simulink model "HD2_QArmTeleopClient"  (R2018a)
settings: Solver=ode1  StartTime=0.0  StopTime=inf  FixedStep=0.001  RelTol=1e-3  EnableMultiTasking=on
model workspace (MAT data in the model file):
  ErrTol = Simulink.Parameter
  ErrTol.Value = 0.0001
  ErrTol.DataType = 'auto'
  ErrTol.Dimensions = [1 1]
undefined symbols (not defined in the file): gcbh, Host, JPEG, video_display_show, Visualization
libraries: quarc_library x15, simulink x6, simulink_extras x3
settings Model: SimulationMode=external  ExtModeTrigDuration=10000  Creator=glai  LastModifiedBy=QuanserGraphics
settings SolverCC: PositivePriorityOrder=on
settings RTWCC: SystemTargetFile=quarc_win64.tlc  TemplateMakefile=quarc_default_tmf  Description=QUARC Win64 Target Using Toolchain  Toolchain=QUARC win64 | nmake (64-bit Windows)  BuildConfiguration=Faster Runs
settings CodeAppCC: StateflowObjectComments=on
settings STFCustomTargetCC: TargetLangStandard=C99 (ISO)  ConcurrentExecutionCompliant=on  UseToolchainInfoCompliant=on  SystemTargetFile=quarc_win64.tlc
settings GRTTargetCC: ParMdlRefBuildCompliant=off  CompOptLevelCompliant=off  CombineOutputUpdateFcns=off  MatFileLogging=off  CPPClassGenCompliant=off  GRTInterface=on  ExtMode=on  ExtModeMexFile=quarc_comm  ExtModeMexArgs='-w -d %d -uri %u -URI_SHMEM shmem://HD2_DRIVER_PY:0','tcpip://localhost:17005'
settings ConfigComp: CovMetricSettings=dswe

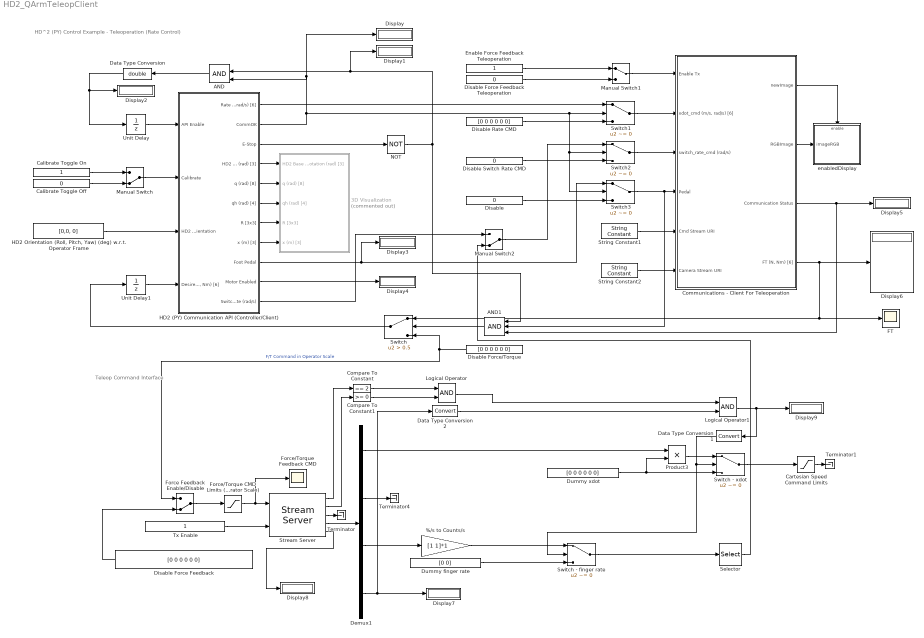
== system HD2_QArmTeleopClient ==
  note: HD^2 (PY) Control Example - Teleoperation (Rate Control)
  note: Teleop Command Interface
  %/s to Counts/s : Gain  Gain=[1 1]*1
  3D Visualization : Subsystem  Commented=on
  AND : Logic  IconShape=distinctive  AllPortsSameDT=off  OutDataTypeStr=boolean
  AND1 : Logic  Inputs=3  IconShape=distinctive  AllPortsSameDT=off  OutDataTypeStr=boolean
  Calibrate Toggle Off : Constant  Value=0
  Calibrate Toggle On : Constant
  Cartesian Speed Command Limits : Saturate  UpperLimit=[0.254 0.254 0.254 0.06 0.06 0.06]  LowerLimit=-1*[0.254 0.254 0.254 0.06 0.06 0.06]
  Communications - Client For Teleoperation : Subsystem
  Compare To Constant : simulink/Logic and Bit Operations/Compare To Constant  relop===  const=2  OutDataTypeStr=boolean
  Compare To Constant1 : simulink/Logic and Bit Operations/Compare To Constant  relop=>=  const=0  OutDataTypeStr=boolean
  Data Type Conversion : DataTypeConversion  OutDataTypeStr=double
  Data Type Conversion1 : DataTypeConversion
  Data Type Conversion2 : DataTypeConversion
  Demux1 : Demux  Outputs=[6 6 1 1]
  Disable : Constant  Value=0
  Disable Force Feedback : Constant  Value=[0 0 0 0 0 0]
  Disable Force Feedback Teleoperation : Constant  Value=0
  Disable Force/Torque : Constant  Value=[0 0 0 0 0 0]
  Disable Rate CMD : Constant  Value=[0 0 0 0 0 0]
  Disable Switch Rate CMD : Constant  Value=0
  Display{,1..9} (10 alike) : Display
      Display settings: Decimation=100
      Display1 settings: Decimation=100
      Display2 settings: Decimation=100
      Display3 settings: Decimation=100
      Display4 settings: Decimation=100
      Display5 settings: Decimation=100
      Display7 settings: Decimation=100
      Display8 settings: Decimation=100
      Display9 settings: Decimation=100
  Dummy finger rate : Constant  Value=[0 0]
  Dummy xdot : Constant  Value=[0 0 0 0 0 0]
  Enable Force Feedback Teleoperation : Constant
  FT : Scope
  Force Feedback Enable/Disable : ManualSwitch  CurrentSetting=0
  Force/Torque CMD Limits (Operator Scale) : Saturate  UpperLimit=[3 3 3 0.2 0.2 0.2]  LowerLimit=-1*[3 3 3 0.2 0.2 0.2]
  Force/Torque Feedback CMD : Scope
  HD2 (PY) Communication API (Controller/Client) : Subsystem
  "HD2 Orientation (Roll, Pitch, Yaw) (deg) w.r.t. Operator Frame" : Constant  Value=[0,0, 0]
  Logical Operator : Logic  AllPortsSameDT=off  OutDataTypeStr=boolean
  Logical Operator1 : Logic  AllPortsSameDT=off  OutDataTypeStr=boolean
  Manual Switch : ManualSwitch  CurrentSetting=0
  Manual Switch1 : ManualSwitch
  Manual Switch2 : ManualSwitch  CurrentSetting=0
  NOT : Logic  Operator=NOT  IconShape=distinctive  AllPortsSameDT=off  OutDataTypeStr=boolean
  Product3 : Product
  Selector : Selector  InputPortWidth=2  IndexOptions=Index vector (dialog)  Indices=[1]  OutputSizes=1
  Stream Server : quarc_library/Communications/Basic/Stream Server  uri_source=Specify via dialog (do not evaluate)  uri=tcpip://localhost:18008  send_buffer_size=1460  receive_buffer_size=1460  byte_order=little endian (Intel - LSB first)  optimization=Minimum latency  send_options=Send most recent data  receive_options=Receive most recent data  default_value=zeros(1,14)  sample_time=qc_get_step_size  active=off  implementation=Use blocking I/O in a separate thread  send_fifo_size=1000  receive_fifo_size=1000  send_priority=0  receive_priority=0  send_dimensions=off  receive_dimensions=off  max_dimensions=-1  data_type=Inherited via back propagation  type_expr=BusObject
      settings: AttributesFormatString="\"tcpip://localhost:18008\""
  String Constant1 : quarc_library/Strings/String Constant  string_value=tcpip://localhost:18018  evaluate_string=off  string_type=text  max_length=80  sample_time=inf  variable_size=off
      settings: AttributesFormatString="\"tcpip://localhost:18018\""  SourceProductName=QUARC Targets
  String Constant2 : quarc_library/Strings/String Constant  string_value=tcpip://localhost:18025  evaluate_string=off  string_type=text  max_length=80  sample_time=inf  variable_size=off
      settings: AttributesFormatString="\"tcpip://localhost:18025\""  SourceProductName=QUARC Targets
  Switch : Switch  Criteria=u2 > Threshold  Threshold=0.5
  Switch - finger rate : Switch  Criteria=u2 ~= 0
  Switch - xdot : Switch  Criteria=u2 ~= 0
  Switch1 : Switch  Criteria=u2 ~= 0  Threshold=0.5
  Switch2 : Switch  Criteria=u2 ~= 0  Threshold=0.5
  Switch3 : Switch  Criteria=u2 ~= 0  Threshold=0.5
  Terminator : Terminator
  Terminator1 : Terminator
  Terminator4 : Terminator
  Tx Enable : Constant
  Unit Delay : UnitDelay  SampleTime=-1
  Unit Delay1 : UnitDelay  SampleTime=-1
  enabledDisplay : Subsystem  TreatAsAtomicUnit=on
  wires:
  Selector/1 -> Manual Switch2/2
  Demux1/4 -> Display7/1, Data Type Conversion2/1
  Disable Force/Torque/1 -> Switch/3, Force Feedback Enable/Disable/1  "F/T Command in Operator Scale"
  Disable Force Feedback/1 -> Force Feedback Enable/Disable/2
  Data Type Conversion/1 -> Unit Delay/1, Display2/1
  Switch2/1 -> Communications - Client For Teleoperation/3(switch_rate_cmd (rad/s))
  Stream Server/4 -> Demux1/1
  Disable Switch Rate CMD/1 -> Switch2/3
  HD2 (PY) Communication API (Controller/Client)/11(Switch Rate (rad/s)) -> Manual Switch2/1
  Unit Delay/1 -> HD2 (PY) Communication API (Controller/Client)/1(API Enable)
  Switch - finger rate/1 -> Selector/1
  HD2 (PY) Communication API (Controller/Client)/3(E-Stop) -> NOT/1
  HD2 (PY) Communication API (Controller/Client)/7(R [3x3]) -> 3D Visualization/4(R [3x3])
  Manual Switch2/1 -> Switch2/1
  Force/Torque CMD Limits (Operator Scale)/1 -> Force/Torque Feedback CMD/1, Stream Server/1
  AND/1 -> Data Type Conversion/1
  Data Type Conversion2/1 -> Logical Operator1/2
  Logical Operator/1 -> Logical Operator1/1
  Stream Server/2 -> Compare To Constant1/1
  Data Type Conversion1/1 -> Switch - finger rate/2, Switch - xdot/2
  Dummy finger rate/1 -> Switch - finger rate/3
  Stream Server/5 -> Display8/1
  Communications - Client For Teleoperation/4("FT (N, Nm) [6]") -> Display6/1, FT/1, Switch/1
  Compare To Constant1/1 -> Logical Operator/2
  HD2 (PY) Communication API (Controller/Client)/4(HD2 Rotation (rad) [3]) -> 3D Visualization/1(HD2 Base Rotation (rad) [3])
  %/s to Counts/s/1 -> Switch - finger rate/1
  Dummy xdot/1 -> Product3/2, Switch - xdot/3
  HD2 (PY) Communication API (Controller/Client)/8(x (m) [3]) -> 3D Visualization/5(x (m) [3])
  Demux1/1 -> Product3/1
  Disable Rate CMD/1 -> Switch1/3
  Cartesian Speed Command Limits/1 -> Terminator1/1
  Force Feedback Enable/Disable/1 -> Force/Torque CMD Limits (Operator Scale)/1
  HD2 (PY) Communication API (Controller/Client)/5(q (rad) [8]) -> 3D Visualization/2(q (rad) [8])
  Product3/1 -> Switch - xdot/1
  Switch/1 -> Unit Delay1/1
  Communications - Client For Teleoperation/3(Communication Status) -> AND1/3, Display5/1
  AND1/1 -> Switch/2
  Stream Server/3 -> Terminator/1
  HD2 (PY) Communication API (Controller/Client)/10(Motor Enabled) -> Display4/1
  Compare To Constant/1 -> Logical Operator/1
  Unit Delay1/1 -> HD2 (PY) Communication API (Controller/Client)/4("Desired FT (N, Nm) [6]")
  Manual Switch1/1 -> Communications - Client For Teleoperation/1(Enable Tx)
  Switch1/1 -> Communications - Client For Teleoperation/2("xdot_cmd (m/s, rad/s) [6]")
  Switch - xdot/1 -> Cartesian Speed Command Limits/1
  HD2 (PY) Communication API (Controller/Client)/6(qh (rad) [4]) -> 3D Visualization/3(qh (rad) [4])
  HD2 (PY) Communication API (Controller/Client)/9(Foot Pedal) -> Display3/1, Switch3/1
  Logical Operator1/1 -> Display9/1, Data Type Conversion1/1
  Disable/1 -> Switch3/3
  HD2 (PY) Communication API (Controller/Client)/2(CommOK) -> AND/2, Display/1, Switch3/2, Switch2/2, Switch1/2
  Tx Enable/1 -> Stream Server/2
  Enable Force Feedback Teleoperation/1 -> Manual Switch1/1
  String Constant1/1 -> Communications - Client For Teleoperation/5(Cmd Stream URI)
  Demux1/2 -> Terminator4/1
  Disable Force Feedback Teleoperation/1 -> Manual Switch1/2
  NOT/1 -> AND1/1, AND/1, Display1/1
  Demux1/3 -> %/s to Counts/s/1
  HD2 (PY) Communication API (Controller/Client)/1("Rate CMD (m/s, rad/s) [6]") -> Switch1/1
  Stream Server/1 -> Compare To Constant/1
  Switch3/1 -> AND1/2, Communications - Client For Teleoperation/4(Pedal)
  String Constant2/1 -> Communications - Client For Teleoperation/6(Camera Stream URI)
  Calibrate Toggle On/1 -> Manual Switch/1
  Calibrate Toggle Off/1 -> Manual Switch/2
  Manual Switch/1 -> HD2 (PY) Communication API (Controller/Client)/2(Calibrate)
  "HD2 Orientation (Roll, Pitch, Yaw) (deg) w.r.t. Operator Frame"/1 -> HD2 (PY) Communication API (Controller/Client)/3(HD2 Orientation)
  Communications - Client For Teleoperation/2(RGBImage) -> enabledDisplay/1(imageRGB)
  Communications - Client For Teleoperation/1(newImage) -> enabledDisplay/Enable

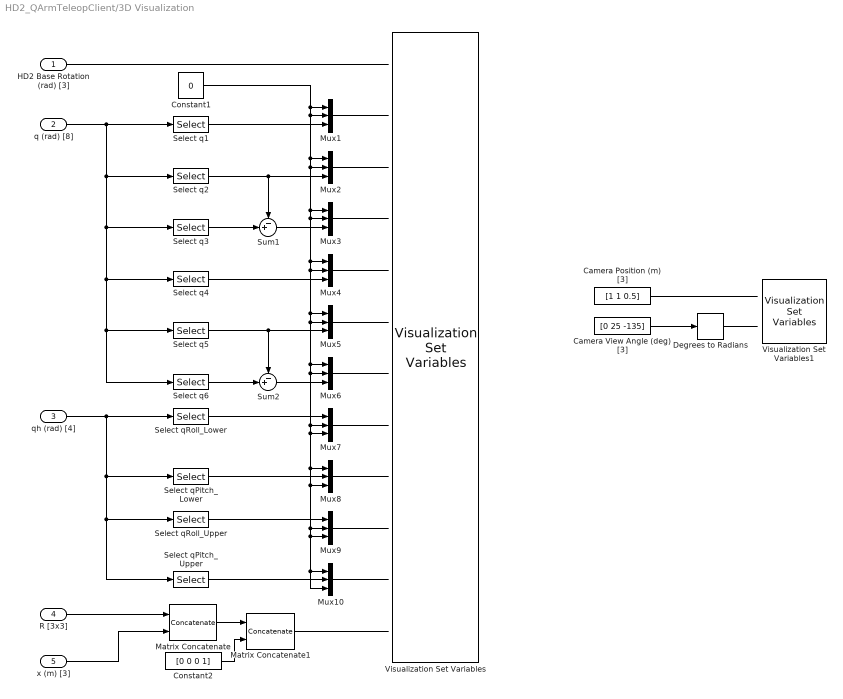
== system HD2_QArmTeleopClient/3D Visualization ==
  HD2 Base Rotation (rad) [3] : Inport
  q (rad) [8] : Inport  Port=2
  qh (rad) [4] : Inport  Port=3
  R [3x3] : Inport  Port=4
  x (m) [3] : Inport  Port=5
  Camera Position (m) [3] : Constant  Value=[1 1 0.5]  VectorParams1D=off
  Camera View Angle (deg) [3] : Constant  Value=[0 25 -135]  VectorParams1D=off
  Constant1 : Constant  Value=0
  Constant2 : Constant  Value=[0 0 0 1]  VectorParams1D=off
  Degrees to Radians : simulink_extras/Transformations/Degrees to Radians
  Matrix Concatenate : Concatenate  Mode=Multidimensional array  ConcatenateDimension=2
  Matrix Concatenate1 : Concatenate  Mode=Multidimensional array
  Mux{1..10} (10 alike) : Mux  Inputs=3
  Select q1 : Selector  InputPortWidth=8  IndexOptions=Index vector (dialog)  Indices=[1]  OutputSizes=1
  Select q2 : Selector  InputPortWidth=8  IndexOptions=Index vector (dialog)  Indices=[2]  OutputSizes=1
  Select q3 : Selector  InputPortWidth=8  IndexOptions=Index vector (dialog)  Indices=[3]  OutputSizes=1
  Select q4 : Selector  InputPortWidth=8  IndexOptions=Index vector (dialog)  Indices=[4]  OutputSizes=1
  Select q5 : Selector  InputPortWidth=8  IndexOptions=Index vector (dialog)  Indices=[5]  OutputSizes=1
  Select q6 : Selector  InputPortWidth=8  IndexOptions=Index vector (dialog)  Indices=[6]  OutputSizes=1
  Select qPitch_Lower : Selector  InputPortWidth=4  IndexOptions=Index vector (dialog)  Indices=[2]  OutputSizes=1
  Select qPitch_Upper : Selector  InputPortWidth=4  IndexOptions=Index vector (dialog)  Indices=[4]  OutputSizes=1
  Select qRoll_Lower : Selector  InputPortWidth=4  IndexOptions=Index vector (dialog)  Indices=[1]  OutputSizes=1
  Select qRoll_Upper : Selector  InputPortWidth=4  IndexOptions=Index vector (dialog)  Indices=[3]  OutputSizes=1
  Sum1 : Sum  Inputs=-+|
  Sum2 : Sum  Inputs=-+|
  Visualization Set Variables : quarc_library/User Interface/Visualization/Visualization Set Variables  object_name=Visualization-1  offset="[  ]"  data_type="[  ]"  length="[  ]"  sample_time=visualization_get_frame_period  actor_name={'RefFrame.Base/Orientation';'RefFrame.Upper.J0/Orientation';'RefFrame.Upper.J1/Orientation';'RefFrame.Upper.J2/Orientation';'RefFrame.Lower.J0/Orientation';'RefFrame.Lower.J1/Orientation';'RefFrame.Lower.J2/Orientation';'RefFrame.Upper.qRoll/Orientation';'RefFrame.Upper.qPitch/Orientation';'RefFrame.Lower.qRoll/Orientation';'RefFrame.Lower.qPitch/Orientation';'RefFrame.Handle.EE/Transform'}
      settings: AttributesFormatString=(%<object_name>)  SourceProductName=QUARC Targets
  Visualization Set Variables1 : quarc_library/User Interface/Visualization/Visualization Set Variables  object_name=Visualization-1  offset="[  ]"  data_type="[  ]"  length="[  ]"  sample_time=visualization_get_frame_period  actor_name={'actor.camera/Position';'actor.camera/Orientation'}
      settings: AttributesFormatString=(%<object_name>)  SourceProductName=QUARC Targets
  wires:
  Sum2/1 -> Mux6/3
  Select q6/1 -> Sum2/2
  Matrix Concatenate/1 -> Matrix Concatenate1/1
  Constant1/1 -> Mux2/2, Mux3/1, Mux4/1, Mux5/1, Mux6/1, Mux8/1, Mux9/2, Mux10/1, Mux10/3, Mux9/3, Mux8/3, Mux7/3, Mux7/2, Mux6/2, Mux5/2, Mux4/2, Mux3/2, Mux2/1, Mux1/2, Mux1/1
  Sum1/1 -> Mux3/3
  Select q2/1 -> Sum1/1, Mux2/3
  Select q3/1 -> Sum1/2
  Constant2/1 -> Matrix Concatenate1/2
  Select q4/1 -> Mux4/3
  Select qRoll_Upper/1 -> Mux9/1
  Select q1/1 -> Mux1/3
  Select q5/1 -> Sum2/1, Mux5/3
  Select qRoll_Lower/1 -> Mux7/1
  Select qPitch_Upper/1 -> Mux10/2
  Select qPitch_Lower/1 -> Mux8/2
  x (m) [3]/1 -> Matrix Concatenate/2
  R [3x3]/1 -> Matrix Concatenate/1
  qh (rad) [4]/1 -> Select qPitch_Lower/1, Select qRoll_Upper/1, Select qPitch_Upper/1, Select qRoll_Lower/1
  q (rad) [8]/1 -> Select q2/1, Select q3/1, Select q4/1, Select q5/1, Select q6/1, Select q1/1
  Mux1/1 -> ?
  Mux2/1 -> ?
  Mux3/1 -> ?
  Mux4/1 -> ?
  Mux5/1 -> ?
  Mux6/1 -> ?
  Mux7/1 -> ?
  Mux8/1 -> ?
  Mux9/1 -> ?
  Mux10/1 -> ?
  Matrix Concatenate1/1 -> ?
  HD2 Base Rotation (rad) [3]/1 -> ?
  Camera View Angle (deg) [3]/1 -> Degrees to Radians/1
  Degrees to Radians/1 -> ?
  Camera Position (m) [3]/1 -> ?

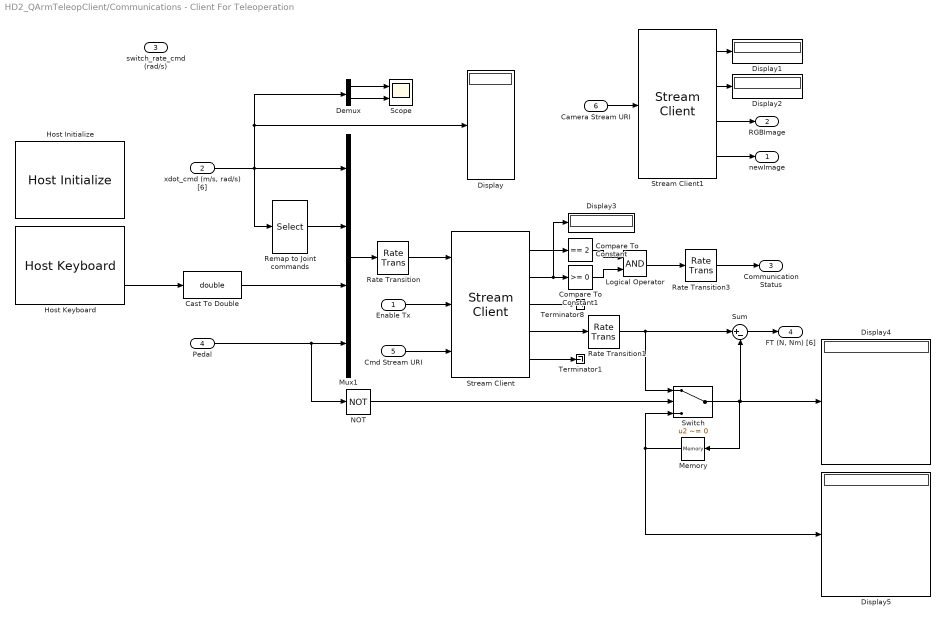
== system HD2_QArmTeleopClient/Communications - Client For Teleoperation ==
  Enable Tx : Inport
  "xdot_cmd (m/s, rad/s) [6]" : Inport  Port=2
  switch_rate_cmd (rad/s) : Inport  Port=3
  Pedal : Inport  Port=4
  Cmd Stream URI : Inport  Port=5
  Camera Stream URI : Inport  Port=6
  Cast To Double : DataTypeConversion  OutDataTypeStr=double
  Compare To Constant : simulink/Logic and Bit Operations/Compare To Constant  relop===  const=2  OutDataTypeStr=uint8
  Compare To Constant1 : simulink/Logic and Bit Operations/Compare To Constant  relop=>=  const=0  OutDataTypeStr=uint8
  Demux : Demux  Outputs=2
  Display{,1..5} (6 alike) : Display
      Display3 settings: Decimation=500
  Host Initialize : quarc_library/Devices/Peripherals/Host/Host Initialize  object_name=Host-1  uri_source=Use external mode communications  uri=tcpip://localhost:18001  send_buffer_size=1000  receive_buffer_size=1000  thread_priority=0  run_client=on  use_window=off  window_position=[]  sample_time=qc_get_step_size  active=on
      settings: SourceProductName=QUARC Targets
  Host Keyboard : quarc_library/Devices/Peripherals/Host/Host Keyboard  object_name=Host-1  virtual_key=[32]  sample_time=qc_get_step_size  enabled=on  debug_mode=off
      settings: SourceProductName=QUARC Targets
  Logical Operator : Logic  AllPortsSameDT=off  OutDataTypeStr=boolean
  Memory : quarc_library/Discrete/Memory  initial_condition=[0,0,0,0,0,0]  sample_time=-1
      settings: SourceProductName=QUARC Targets
  Mux1 : Mux  Inputs=[6 6 1 1]
  NOT : Logic  Operator=NOT  IconShape=distinctive  AllPortsSameDT=off  OutDataTypeStr=boolean
  Rate Transition : RateTransition
  Rate Transition1 : RateTransition
  Rate Transition3 : RateTransition
  Remap to Joint commands : Selector  InputPortWidth=6  IndexOptions=Index vector (dialog)  Indices=[2,1,3,4,5,6]  OutputSizes=1
  Scope : Scope  NumInputPorts=2
  Stream Client : quarc_library/Communications/Basic/Stream Client  uri_source=External input port  uri=tcpip://172.16.191.147:18000  send_buffer_size=1460  receive_buffer_size=1460  byte_order=little endian (Intel - LSB first)  optimization=Minimum latency  send_options=Send most recent data  receive_options=Receive most recent data  default_value=zeros(1,6)  sample_time=qc_get_step_size  active=off  implementation=Use blocking I/O in a separate thread  send_fifo_size=1000  receive_fifo_size=1000  send_priority=0  receive_priority=0  send_dimensions=off  receive_dimensions=off  max_dimensions=-1  data_type=Inherited via back propagation  type_expr=BusObject
  Stream Client1 : quarc_library/Communications/Basic/Stream Client  uri_source=External input port  uri=tcpip://172.16.191.147:18000  send_buffer_size=128  receive_buffer_size=640*480*3  byte_order=little endian (Intel - LSB first)  optimization=Minimum latency  send_options=Do not send data  receive_options=Receive most recent data  default_value=zeros(480, 640, 3)  sample_time=qc_get_step_size  active=off  implementation=Use blocking I/O in a separate thread  send_fifo_size=2  receive_fifo_size=2  send_priority=0  receive_priority=0  send_dimensions=off  receive_dimensions=off  max_dimensions=-1  data_type=uint8  type_expr=BusObject
  Sum : Sum  Inputs=|+-
  Switch : Switch  Criteria=u2 ~= 0
  Terminator1 : Terminator
  Terminator8 : Terminator
  newImage : Outport
  RGBImage : Outport  Port=2
  Communication Status : Outport  Port=3
  "FT (N, Nm) [6]" : Outport  Port=4
  wires:
  "xdot_cmd (m/s, rad/s) [6]"/1 -> Mux1/1, Demux/1, Display/1, Remap to Joint commands/1
  Mux1/1 -> Rate Transition/1
  Rate Transition/1 -> Stream Client/1
  Stream Client/4 -> Rate Transition1/1
  Compare To Constant/1 -> Logical Operator/1
  Compare To Constant1/1 -> Logical Operator/2
  Logical Operator/1 -> Rate Transition3/1
  Stream Client/1 -> Compare To Constant/1
  Stream Client/2 -> Compare To Constant1/1, Display3/1
  Stream Client/3 -> Terminator8/1
  Rate Transition3/1 -> Communication Status/1
  Stream Client/5 -> Terminator1/1
  Enable Tx/1 -> Stream Client/2
  Cmd Stream URI/1 -> Stream Client/3
  Pedal/1 -> NOT/1, Mux1/4
  Remap to Joint commands/1 -> Mux1/2
  Demux/1 -> Scope/1
  Demux/2 -> Scope/2
  Host Keyboard/2 -> Cast To Double/1
  Cast To Double/1 -> Mux1/3
  Stream Client1/1 -> Display1/1
  Camera Stream URI/1 -> Stream Client1/1
  Stream Client1/2 -> Display2/1
  Stream Client1/4 -> newImage/1
  Stream Client1/3 -> RGBImage/1
  NOT/1 -> Switch/2
  Sum/1 -> "FT (N, Nm) [6]"/1
  Rate Transition1/1 -> Sum/1, Switch/1
  Switch/1 -> Display4/1, Sum/2, Memory/1
  Memory/1 -> Display5/1, Switch/3

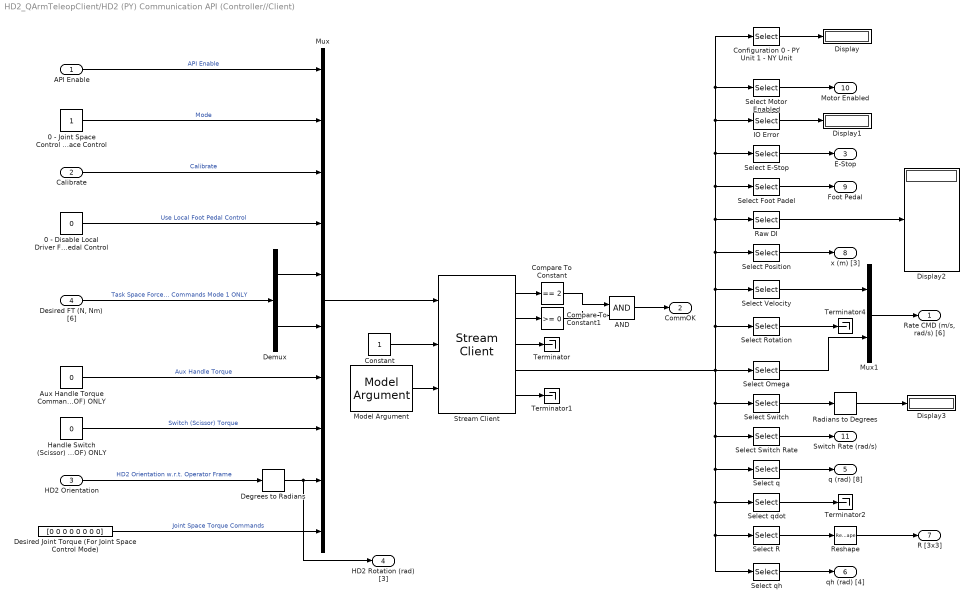
== system HD2_QArmTeleopClient/HD2 (PY) Communication API (Controller//Client) ==
  API Enable : Inport
  Calibrate : Inport  Port=2
  HD2 Orientation : Inport  Port=3
  "Desired FT (N, Nm) [6]" : Inport  Port=4
  0 - Disable Local Driver Foot Pedal Control 1 - Enable Local Driver Foot Pedal Control : Constant  Value=0
  0 - Joint Space Control 1 - Task Space Control : Constant
  AND : Logic  IconShape=distinctive  AllPortsSameDT=off  OutDataTypeStr=boolean
  Aux Handle Torque Command (Nm) Mode 1 (6-DOF or 7-DOF) ONLY : Constant  Value=0
  Compare To Constant : simulink/Logic and Bit Operations/Compare To Constant  relop===  const=2  OutDataTypeStr=boolean
  Compare To Constant1 : simulink/Logic and Bit Operations/Compare To Constant  relop=>=  const=0  OutDataTypeStr=boolean
  Configuration 0 - PY Unit 1 - NY Unit : Selector  InputPortWidth=56  IndexOptions=Index vector (dialog)  Indices=[1]  OutputSizes=1
  Constant : Constant
  Degrees to Radians : simulink_extras/Transformations/Degrees to Radians
  Demux : Demux  Outputs=[3 3]
  Desired Joint Torque (For Joint Space Control Mode) : Constant  Value=[0 0 0 0 0 0 0 0]
  Display{,1..3} (4 alike) : Display
      settings: Decimation=100
  Handle Switch (Scissor) Torque Command (Nm) Mode 1 (7-DOF) ONLY : Constant  Value=0
  IO Error : Selector  InputPortWidth=56  IndexOptions=Index vector (dialog)  Indices=[3]  OutputSizes=1
  Model Argument : quarc_library/Sources/Signals/Model Argument  argument_name=URI_SHMEM  has_value=on  data_type_mode=Specify via dialog  data_type=char  max_length=80  default_value=0  variable_size=off
      settings: AttributesFormatString=(-%<argument_name>)  SourceProductName=QUARC Targets
  Mux : Mux  Inputs=[1 1 1 1 3 3 1 1 3 8]
  Mux1 : Mux  Inputs=2
  Radians to Degrees : simulink_extras/Transformations/Radians to Degrees
  Raw DI : Selector  InputPortWidth=56  IndexOptions=Index vector (dialog)  Indices=[6:13]  OutputSizes=1
  Reshape : Reshape  OutputDimensionality=Customize  OutputDimensions=[3,3]
  Select E-Stop : Selector  InputPortWidth=56  IndexOptions=Index vector (dialog)  Indices=[4]  OutputSizes=1
  Select Foot Padel : Selector  InputPortWidth=56  IndexOptions=Index vector (dialog)  Indices=[5]  OutputSizes=1
  Select Motor Enabled : Selector  InputPortWidth=56  IndexOptions=Index vector (dialog)  Indices=[2]  OutputSizes=1
  Select Omega : Selector  InputPortWidth=56  IndexOptions=Index vector (dialog)  Indices=[23:25]  OutputSizes=1
  Select Position : Selector  InputPortWidth=56  IndexOptions=Index vector (dialog)  Indices=[14:16]  OutputSizes=1
  Select R : Selector  InputPortWidth=56  IndexOptions=Index vector (dialog)  Indices=[44:52]  OutputSizes=1
  Select Rotation : Selector  InputPortWidth=56  IndexOptions=Index vector (dialog)  Indices=[20:22]  OutputSizes=1
  Select Switch : Selector  InputPortWidth=56  IndexOptions=Index vector (dialog)  Indices=[26]  OutputSizes=1
  Select Switch Rate : Selector  InputPortWidth=56  IndexOptions=Index vector (dialog)  Indices=[27]  OutputSizes=1
  Select Velocity : Selector  InputPortWidth=56  IndexOptions=Index vector (dialog)  Indices=[17:19]  OutputSizes=1
  Select q : Selector  InputPortWidth=56  IndexOptions=Index vector (dialog)  Indices=[28:35]  OutputSizes=1
  Select qdot : Selector  InputPortWidth=56  IndexOptions=Index vector (dialog)  Indices=[36:43]  OutputSizes=1
  Select qh : Selector  InputPortWidth=56  IndexOptions=Index vector (dialog)  Indices=[53:56]  OutputSizes=1
  Stream Client : quarc_library/Communications/Basic/Stream Client  uri_source=External input port  uri=tcpip://remotehost:18000  send_buffer_size=2048  receive_buffer_size=2048  byte_order=little endian (Intel - LSB first)  optimization=Minimum latency  send_options=Send most recent data  receive_options=Receive most recent data  default_value=zeros(1,56)  sample_time=qc_get_step_size  active=off  implementation=Use blocking I/O in a separate thread  send_fifo_size=1000  receive_fifo_size=1000  send_priority=0  receive_priority=0  send_dimensions=off  receive_dimensions=off  max_dimensions=-1  data_type=double  type_expr=BusObject
  Terminator{,1..2,4} (4 alike) : Terminator
  "Rate CMD (m/s, rad/s) [6]" : Outport
  CommOK : Outport  Port=2
  E-Stop : Outport  Port=3
  HD2 Rotation (rad) [3] : Outport  Port=4
  q (rad) [8] : Outport  Port=5
  qh (rad) [4] : Outport  Port=6
  R [3x3] : Outport  Port=7
  x (m) [3] : Outport  Port=8
  Foot Pedal : Outport  Port=9
  Motor Enabled : Outport  Port=10
  Switch Rate (rad/s) : Outport  Port=11
  wires:
  AND/1 -> CommOK/1
  Compare To Constant1/1 -> AND/2
  Compare To Constant/1 -> AND/1
  Stream Client/2 -> Compare To Constant1/1
  Stream Client/1 -> Compare To Constant/1
  Model Argument/1 -> Stream Client/3
  Constant/1 -> Stream Client/2
  Stream Client/3 -> Terminator/1
  Stream Client/5 -> Terminator1/1
  Mux/1 -> Stream Client/1
  0 - Joint Space Control 1 - Task Space Control/1 -> Mux/2  "Mode"
  API Enable/1 -> Mux/1  "API Enable"
  HD2 Orientation/1 -> Degrees to Radians/1  "HD2 Orientation w.r.t. Operator Frame"
  Configuration 0 - PY Unit 1 - NY Unit/1 -> Display/1
  Select Motor Enabled/1 -> Motor Enabled/1
  IO Error/1 -> Display1/1
  Select E-Stop/1 -> E-Stop/1
  Stream Client/4 -> Select Switch Rate/1, Select qh/1, Select R/1, Select qdot/1, Select q/1, Select Switch/1, Select Omega/1, Select Rotation/1, Select Velocity/1, Select Position/1, Raw DI/1, Select Foot Padel/1, Select E-Stop/1, Select Motor Enabled/1, Configuration 0 - PY Unit 1 - NY Unit/1, IO Error/1
  Select Foot Padel/1 -> Foot Pedal/1
  Raw DI/1 -> Display2/1
  Select Switch/1 -> Radians to Degrees/1
  Radians to Degrees/1 -> Display3/1
  Select q/1 -> q (rad) [8]/1
  Select R/1 -> Reshape/1
  Select Rotation/1 -> Terminator4/1
  Select qh/1 -> qh (rad) [4]/1
  Reshape/1 -> R [3x3]/1
  Select Position/1 -> x (m) [3]/1
  Select qdot/1 -> Terminator2/1
  Select Switch Rate/1 -> Switch Rate (rad/s)/1
  "Desired FT (N, Nm) [6]"/1 -> Demux/1  "Task Space Force/Torque Commands Mode 1 ONLY"
  Mux1/1 -> "Rate CMD (m/s, rad/s) [6]"/1
  Select Velocity/1 -> Mux1/1
  Select Omega/1 -> Mux1/2
  Calibrate/1 -> Mux/3  "Calibrate"
  Desired Joint Torque (For Joint Space Control Mode)/1 -> Mux/10  "Joint Space Torque Commands"
  Degrees to Radians/1 -> HD2 Rotation (rad) [3]/1, Mux/9
  Handle Switch (Scissor) Torque Command (Nm) Mode 1 (7-DOF) ONLY/1 -> Mux/8  "Switch (Scissor) Torque"
  Aux Handle Torque Command (Nm) Mode 1 (6-DOF or 7-DOF) ONLY/1 -> Mux/7  "Aux Handle Torque"
  Demux/1 -> Mux/5
  Demux/2 -> Mux/6
  0 - Disable Local Driver Foot Pedal Control 1 - Enable Local Driver Foot Pedal Control/1 -> Mux/4  "Use Local Foot Pedal Control"

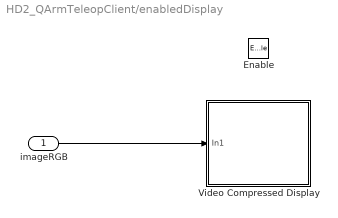
== system HD2_QArmTeleopClient/enabledDisplay ==
  imageRGB : Inport
  Enable : EnablePort  PropagateVarSize=During execution
  Video Compressed Display : Subsystem  LoadFcn=set_param(gcbh, 'UserData', gcb);  StartFcn=video_display_show([gcb, '/Video Display'], 'add', gcb);  mask(Video Compressed Display){algorithm=JPEG, quality=50, sample_time=-1, use_hardware=on}
      mask prompts: algorithm "Compression algorithm:"; quality "Compression quality (0-100):"; sample_time "Sample time (seconds):"; use_hardware "Use hardware acceleration for video display"
      mask help: Displays a video stream on the host, using compression to minimize bandwidth.
      mask init:
      | qc_set_display('Video\nCompressed\nDisplay');
      settings: UndoDeleteFcn=set_param(gcbh, 'UserData', gcb);  OpenFcn=video_display_show([gcb, '/Video Display'], 'show', gcb);  PreDeleteFcn=video_display_show([gcb, '/Video Display'], 'delete');
      settings: CopyFcn=|
      | set_param(gcbh, 'UserData', gcb);
      | set_param(gcbh, 'LinkStatus', 'none');
      settings: NameChangeFcn=|
      | video_display_show([get_param(gcbh, 'UserData'), '/Video Display'], 'rename', [gcb, '/Video Display']);
      | video_display_show([gcb, '/Video Display'], 'add', gcb);
      | set_param(gcbh, 'UserData', gcb);
      mask Help: web(qc_get_block_help_path(gcb));
      mask TypeOptions algorithm: Image Compress/algorithm
      mask TypeOptions quality: Image Compress/quality
      mask TypeOptions sample_time: Video Display/sample_time
      mask TypeOptions use_hardware: Video Display/use_hardware
      mask Display:
      | patch([0.98591 0.98591 0.62618 0.59072 0.56147   0.536   0.536  0.5441 0.56912 0.59207 0.60881 0.62276 0.63527 0.64364  0.6485  0.6485 0.64706 0.64499 0.63662 0.62411 0.61232 0.59837 0.58307 0.56147   0.536   0.536  0.5441  0.5747 0.60953 0.63662 0.67001  0.7034 0.72851 0.75425 0.77927 0.80294 0.82454 0.84119 0.85865 0.87395 0.88574 0.89339  0.8969 0.89969 0.89969 0.89267  0.8816 0.87044 0.85649  0.8384 0.81824 0.80294 0.78764 0.77513 0.76676 0.75776 0.76397 0.77513 0.79178 0.80987 0.82796 0.84326 0.86207 0.98528],[0.18689 0.05522 0.05522 0.05171 0.05171    0.05 0.18338 0.18338 0.19148 0.20435 0.22298 0.24863 0.28589 0.33125 0.38138 0.55139 0.59801 0.63761 0.68189 0.72149 0.74939 0.76694 0.77855 0.79367 0.79952 0.92768 0.92768 0.92768 0.92417 0.92066 0.91364  0.9032 0.89384 0.88106 0.86594 0.85073 0.82634 0.80537 0.77855 0.74363 0.70403 0.65858 0.61079 0.59099 0.41513 0.37202 0.31847 0.29048 0.25556 0.23342  0.2102 0.19382 0.18221 0.17285 0.16943 0.16124  0.1589 0.16241 0.16709 0.17168  0.1787 0.18221 0.18689 0.18689],[0.9,0.90,0.91])
      | patch([0.536 0.52601 0.46823 0.44528 0.41603 0.39101 0.35555 0.33116 0.31451 0.29291  0.2804 0.26717 0.25322 0.23999 0.22406 0.20732 0.19337 0.17528 0.15935 0.14396 0.13217 0.11759 0.10922 0.10085 0.09671 0.09392 0.09041 0.08906 0.08906 0.09464  0.0995 0.10778 0.11894 0.13145 0.14675 0.16349 0.17672 0.19409 0.20732 0.22406 0.23999 0.26159 0.27833 0.29849 0.31793 0.33602 0.35411 0.37085 0.39245 0.41603   0.536   0.536 0.53159 0.46409   0.446 0.42026 0.39587 0.37571 0.36113 0.34925 0.34088 0.33809 0.33809 0.34088 0.34583 0.35627 0.36392 0.38129 0.39587 0.41117 0.42719 0.44672  0.4676 0.48353 0.48353 0.52394   0.536],[0.05 0.04829 0.04712 0.04712 0.04829 0.05063 0.05405 0.05873 0.06107 0.06692 0.07043 0.07619 0.08087 0.08672 0.09482 0.10652 0.11696 0.13325  0.1508 0.17168 0.19499 0.22415 0.25439 0.28472 0.31379 0.35456 0.38489 0.41513 0.58055 0.63878 0.68774 0.72149 0.75641 0.78089 0.80537 0.82859 0.84029 0.85658 0.86594 0.87404  0.8834 0.89267 0.90086 0.90788 0.91247 0.91832 0.92066   0.923 0.92651 0.92768 0.92768 0.79952 0.79952 0.79952 0.79718 0.78899 0.77153 0.75056 0.72149 0.68072 0.62249  0.5549 0.41396 0.37085 0.33242 0.28121 0.25205 0.22181 0.20552 0.19499 0.18572 0.18221 0.17753 0.17636 0.17753  0.1787  0.1787],[0.9,0.90,0.91])
      | disp('Video\nCompressed\nDisplay');
  wires:
  imageRGB/1 -> Video Compressed Display/1(In1)

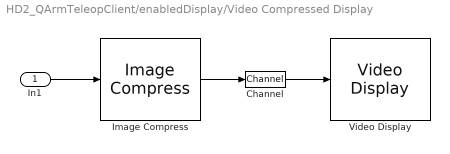
== system HD2_QArmTeleopClient/enabledDisplay/Video Compressed Display ==
  In1 : Inport
  Channel : quarc_library/Signal Routing/Channel  channel=0  buffer_size=1
  Image Compress : quarc_library/Image Processing/Generic/Image Compress  algorithm=JPEG  source=Internal dialog parameter  quality=quality  output_dim=-1
  Video Display : quarc_library/Multimedia/Video Display  Tag=HD2_QArmTeleopClient/enabledDisplay/Video Compressed Display/Video Display  sample_time=sample_time  use_hardware=on
  wires:
  Image Compress/1 -> Channel/1
  In1/1 -> Image Compress/1
  Channel/1 -> Video Display/1
